simulink model "speedgoat_test_SN5659_R2021b_IO133"  (R2021b)
settings: Solver=FixedStepDiscrete  StartTime=0.0  StopTime=20  RelTol=1e-3
PreLoadFcn:
  | Ts_IO107 = 0.001;
  | Ts_IO107 = 0.001;
  | Ts_IO133 = 0.001
  | 
  | Ts_IO204 = 0.001;
  | 
  | 
  | Ts_IO503 = 0.01;
  | 
  | ts_IO612 = 1e-3;
  | Ts_IO682 = 0.005;
  | Ts_IO941 = 0.01;
InitFcn:
  | Ts_IO107 = 0.001;
  | Ts_IO107 = 0.001;
  | Ts_IO133 = 0.001
  | 
  | Ts_IO204 = 0.001;
  | 
  | 
  | Ts_IO503 = 0.01;
  | 
  | ts_IO612 = 1e-3;
  | Ts_IO682 = 0.005;
  | Ts_IO941 = 0.01;
StopFcn:
  | if isfile(['sdi_view_',bdroot,'.mldatx'])
  |  Simulink.sdi.clearPreferences();
  |  Simulink.sdi.view();
  |  pause(3);
  |  Simulink.sdi.loadView(['sdi_view_',bdroot,]);
  | end
libraries: speedgoatlib_IO133 x5, simulink x1
settings Model: Creator=yannick.orgas  LastModifiedBy=ACH
settings SolverCC: ConcurrentTasks=on  AlgebraicLoopSolver=TrustRegion  PositivePriorityOrder=on
settings DataIOCC: LimitDataPoints=on  SaveFormat=StructureWithTime
settings OptimizationCC: BlockReduction=off  OptimizeBlockIOStorage=off
settings DebuggingCC: TasksWithSamePriorityMsg=none  UnconnectedInputMsg=none  UnconnectedOutputMsg=none  UnconnectedLineMsg=none  SFMachineParentedDataDiag=warning
settings HardwareCC: ProdBitPerLong=64  ProdLongLongMode=on  ProdHWDeviceType=Intel->x86-64 (Linux 64)
settings RTWCC: Description=Simulink Real-Time  SystemTargetFile=slrealtime.tlc  TemplateMakefile=slrealtime_default_tmf  Toolchain=Simulink Real-Time Toolchain  BuildConfiguration=Faster Runs  CodeExecutionProfiling=on  TargetLang=C++
settings SimulinkRealTimeTargetCC: UseGCCFastMath=on

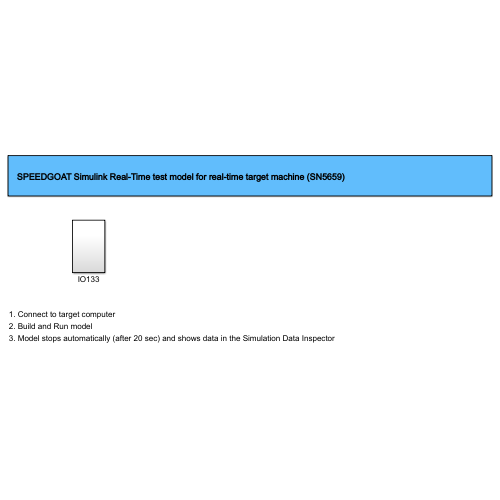
[thumbnail: Simulink's stored preview of the top-level diagram]
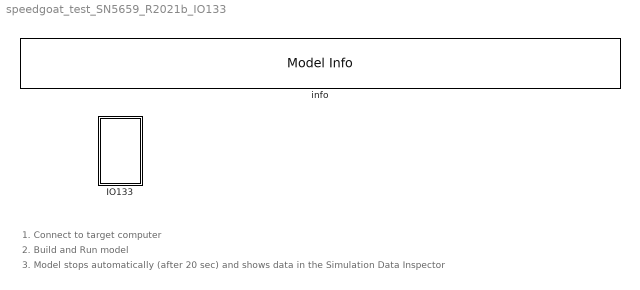
== system speedgoat_test_SN5659_R2021b_IO133 ==
  note: 1. Connect to target computer
  note: 2. Build and Run model
  note: 3. Model stops automatically (after 20 sec) and shows data in the Simulation Data Inspector
  IO133 : Subsystem
  info : simulink/Model-Wide Utilities/Model Info  Frame=on  DisplayStringWithTags=SPEEDGOAT Simulink Real-Time test model for real-time target machine (SN5659)  HorizontalTextAlignment=Left  LeftAlignmentValue=0.02

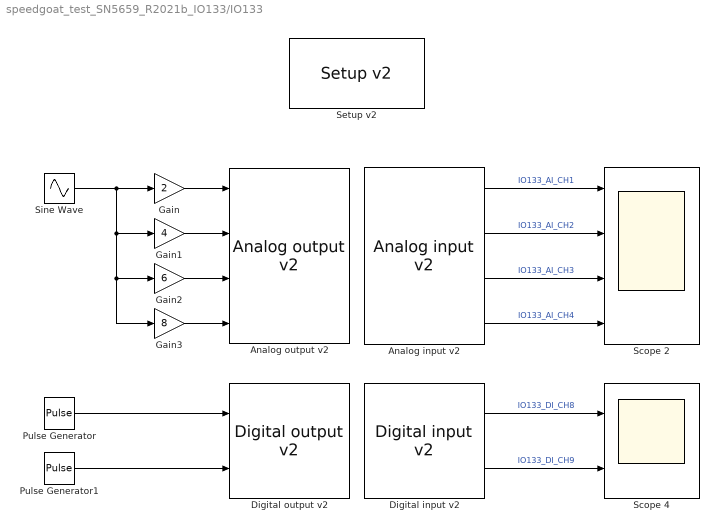
== system speedgoat_test_SN5659_R2021b_IO133/IO133 ==
  "Analog input v2 " : speedgoatlib_IO133/Analog input v2   parModuleId=1  parSampleTime=Ts_IO133  parPciSlot=-1  parAdcChannels=[1 2 3 4]  parAdcVoltageRange=[2 2]  parAdcOversamplRate=[1 1]  parAdcContSampling=0  parAdcDmaEnable=0  parAdcActiveDmaDevices=[1 1]  parAdcFrameSize=100
      settings: SourceProductName=Simulink Real-Time: Speedgoat I/O Driver Library
  "Analog output v2 " : speedgoatlib_IO133/Analog output v2   parModuleId=1  parSampleTime=Ts_IO133  parPciSlot=-1  parDacChannels=[1 2 3 4]  parDacVoltageRange=[4 4 6 6 5 5 5 5]  parDacInitValues=[0 0 0 0]  parDacReset=[1 1 1 1]  parDacSyncOut=1  parDacDmaEnable=0  parDacActiveDmaDevices=[1 1]  parDacDmaLatency=2  parDacFrameSize=100
      settings: SourceProductName=Simulink Real-Time: Speedgoat I/O Driver Library
  "Digital input v2 " : speedgoatlib_IO133/Digital input v2   parModuleId=1  parSampleTime=Ts_IO133  parPciSlot=-1  parDiChannels=[8 9]
      settings: SourceProductName=Simulink Real-Time: Speedgoat I/O Driver Library
  "Digital output v2 " : speedgoatlib_IO133/Digital output v2   parModuleId=1  parSampleTime=Ts_IO133  parPciSlot=-1  parDoChannels=[1 2]  parDoInitValues=[0 0]  parDoReset=[1 1]
      settings: SourceProductName=Simulink Real-Time: Speedgoat I/O Driver Library
  Gain : Gain  Gain=2
  Gain1 : Gain  Gain=4
  Gain2 : Gain  Gain=6
  Gain3 : Gain  Gain=8
  Pulse Generator : DiscretePulseGenerator  Period=20  PulseWidth=5  SampleTime=Ts_IO133
  Pulse Generator1 : DiscretePulseGenerator  Period=20  PulseWidth=10  SampleTime=Ts_IO133
  "Scope 2 " : Scope  NumInputPorts=4
  "Scope 4 " : Scope  NumInputPorts=2
  "Setup v2 " : speedgoatlib_IO133/Setup v2   parPciSlot=-1  parModuleId=1  parInterModuleSync=None  parConvClockBaseRate=20MHz  parConvClock1Divider=20000  parConvClock2Divider=20000  parFrameTriggerEnable=off  parFrameTriggerDivider=10  parConvClock1BaseRate=1  parConvClock2BaseRate=1  parFrameTriggerClock=1  parAdcChannels=1:4  parAdcRange1=+-10V  parAdcRange2=+-10V  parAdcVoltageRange=[2 2]  parAdcOversampling1=None  parAdcOversampling2=None  parAdcOversamplRate=[1 1]  parAdcAutoCorrection=on  parAdcContSampling=off  parAdcDmaEnable=off  parAdcDmaClock=Clock 1  parAdcFrameSize_=100  parAdcSampleTime_=-1  parAdcActiveDmaDevices=[1 1]  parAdcFrameTriggerEnable=0  parAdcFrameSize=100  parAdcSampleTime=0.1  parDacChannels=1:4  parDacInitValues=0  parDacReset=1  parDacRange1=+-5V  parDacRange2=+-5V  parDacRange3=+-10.8V  parDacRange4=+-10.8V  parDacRange5=+-10V  parDacRange6=+-10V  parDacRange7=+-10V  parDacRange8=+-10V  parDacVoltageRange=[4 4 6 6 5 5 5 5]  parDacAutoCorrection=on  parDacSyncOut=on  parDacDmaEnable=off  parDacDmaLatency=Until next frame  parDacDmaClock=Clock 1  parDacFrameSize_=100  parDacSampleTime_=-1  parDacActiveDmaDevices=[1 1]  parDacFrameTriggerEnable=0  parDacFrameSize=100  parDacSampleTime=0.1  parDoChannels=1:2  parDoInitValues=0  parDoReset=1  parDiChannels=8:9  parDiDebounceEnable=off  parDiDebounceTime=0  parDiDebounceValue=0  parDioPullRefFront=Pull-up 3.3V  parDioPullRefRear=Floating
      settings: SourceProductName=Simulink Real-Time: Speedgoat I/O Driver Library
  Sine Wave : Sin  Frequency=50  SampleTime=0
  wires:
  Pulse Generator/1 -> "Digital output v2 "/1
  Gain1/1 -> "Analog output v2 "/2
  Gain/1 -> "Analog output v2 "/1
  Gain3/1 -> "Analog output v2 "/4
  Gain2/1 -> "Analog output v2 "/3
  Sine Wave/1 -> Gain/1, Gain1/1, Gain2/1, Gain3/1
  Pulse Generator1/1 -> "Digital output v2 "/2
  "Analog input v2 "/1 -> "Scope 2 "/1  "IO133_AI_CH1"
  "Analog input v2 "/2 -> "Scope 2 "/2  "IO133_AI_CH2"
  "Analog input v2 "/3 -> "Scope 2 "/3  "IO133_AI_CH3"
  "Analog input v2 "/4 -> "Scope 2 "/4  "IO133_AI_CH4"
  "Digital input v2 "/1 -> "Scope 4 "/1  "IO133_DI_CH8"
  "Digital input v2 "/2 -> "Scope 4 "/2  "IO133_DI_CH9"
